simulink subsystem "Torque_Vectoring"  (R2023b)
settings: Solver=VariableStepAuto  StartTime=0.0  StopTime=10.0  RelTol=1e-3
undefined symbols (not defined in the file): chassis, powertrain, sim, suspension, tvs
libraries: simulink x1
settings Model: Creator=Inver  LastModifiedBy=Inver
settings SFSimCC: SimCustomHeaderCode="#include \"simplex.h\""  SimUserSources=Code_Generation_Project/simplex.c

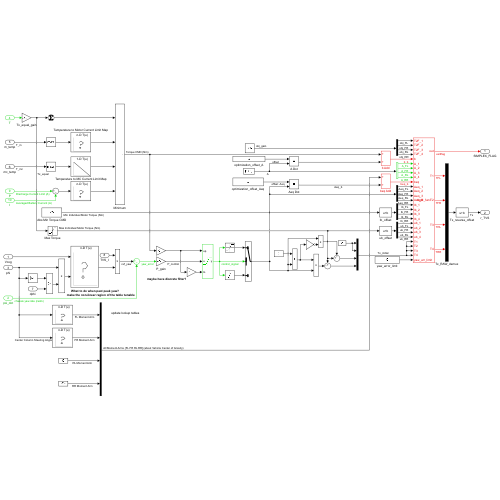
[thumbnail: Simulink's stored preview of the top-level diagram]
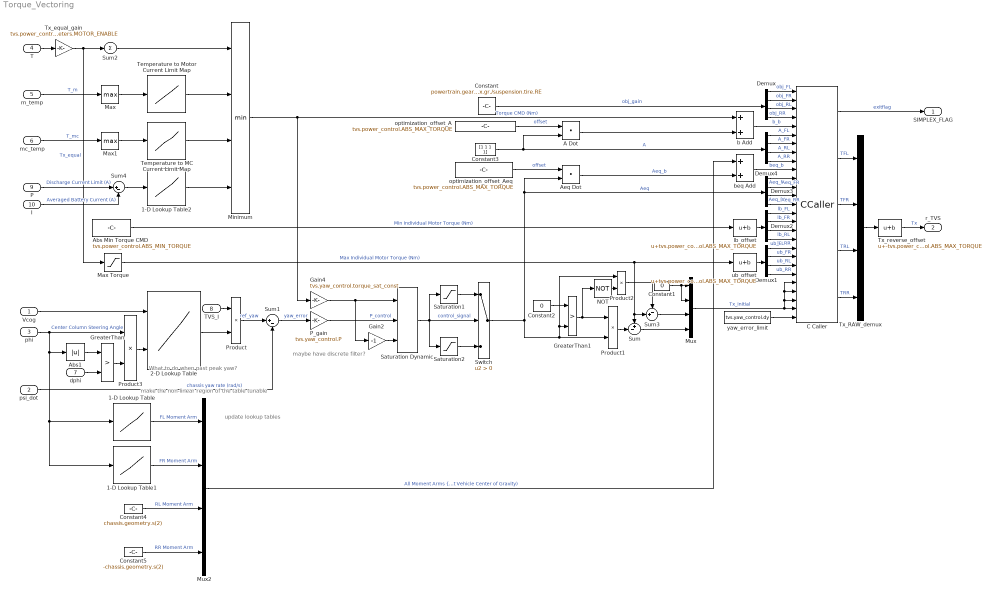
== system Torque_Vectoring ==
  note: make the non-linear region of the table tunable
  note: update lookup tables
  note: maybe have discrete filter?
  note: What to do when past peak yaw?
  Vcog : Inport
  psi_dot : Inport  Port=2  OutDataTypeStr=double  LockScale=on
  phi : Inport  Port=3
  T : Inport  Port=4  OutDataTypeStr=double  LockScale=on
  m_temp : Inport  Port=5
  mc_temp : Inport  Port=6
  dphi : Inport  Port=7
  TVS_I : Inport  Port=8
  P : Inport  Port=9  OutDataTypeStr=double  LockScale=on
  I : Inport  Port=10  OutDataTypeStr=double  LockScale=on
  1-D Lookup Table : Lookup_n-D  NumberOfTableDimensions=1  BreakpointsForDimension1=suspension.steering.theta_sweep  Table=suspension.steering.Aeq_left  ExtrapMethod=Clip  InternalRulePriority=Speed  RndMeth=Simplest
  1-D Lookup Table1 : Lookup_n-D  NumberOfTableDimensions=1  BreakpointsForDimension1=suspension.steering.theta_sweep  Table=suspension.steering.Aeq_right  ExtrapMethod=Clip  InternalRulePriority=Speed  RndMeth=Simplest
  1-D Lookup Table2 : Lookup_n-D  NumberOfTableDimensions=1  LookupTableObject=''  BreakpointsForDimension1=[5 0]  BreakpointsForDimension1FirstPoint=10  BreakpointsForDimension2FirstPoint=10  BreakpointsForDimension1Spacing=12  BreakpointsForDimension2Spacing=12  IndexSearchMethod=Evenly spaced points  Table=[tvs.power_control.ABS_MAX_TRQ_CMD 0]  InterpMethod=Flat  DiagnosticForOutOfRangeInput=Error  InternalRulePriority=Speed  RndMeth=Simplest
  2-D Lookup Table : Lookup_n-D  BreakpointsForDimension1=tvs.yaw_control.max_v_bp  BreakpointsForDimension2=[-fliplr(tvs.yaw_control.max_s_bp(2:end)) tvs.yaw_control.max_s_bp]  Table=[-flipud(tvs.yaw_control.max_yaw_table_ref(2:end,:)); tvs.yaw_control.max_yaw_table_ref]'  ExtrapMethod=Clip  InternalRulePriority=Speed  RndMeth=Simplest
      settings: InputPortMap=u0,u1
  A Dot : DotProduct  OutDataTypeStr=double
  Abs Min Torque CMD : Constant  Value=tvs.power_control.ABS_MIN_TORQUE  OutDataTypeStr=double
  Abs1 : Abs  SaturateOnIntegerOverflow=off
  Aeq Dot : DotProduct  OutDataTypeStr=double
  C Caller : CCaller  FunctionName=bigM_func  PortSpecificationStruct="%)30     .    N\"X   8    (     @         %    \"    !P    !     0         %  0 \"0    $    _    07)G3F%M90  4&]R=$YA;64 4V-O<&4     26YD97@     5'EP90      4VEZ90      27-';&]B86P   X    P    !@    @    $          4    (     0    ,    !         !   P!O=70 #@   #     &    \"     0         !0    @    !     P    $         $  # &]U=  .    .     8    (    !          %    \"     $    &     0         0  ...(+15750 chars)"
  Constant : Constant  Value=powertrain.gearbox.gr./suspension.tire.RE
  Constant1 : Constant  Value=0
  Constant2 : Constant  Value=0
  Constant3 : Constant  Value=[1 1 1 1]
  Constant4 : Constant  Value=chassis.geometry.s(2)  OutDataTypeStr=Inherit: Inherit via back propagation
  Constant5 : Constant  Value=-chassis.geometry.s(2)  OutDataTypeStr=Inherit: Inherit via back propagation
  Demux{,1..4} (5 alike) : Demux
  Gain2 : Gain  Gain=-1
  Gain4 : Gain  Gain=tvs.yaw_control.torque_sat_const
  GreaterThan : RelationalOperator  Operator=>  OutDataTypeStr=boolean  RndMeth=Simplest  InputSameDT=off
  GreaterThan1 : RelationalOperator  Operator=>  OutDataTypeStr=boolean  RndMeth=Simplest  InputSameDT=off
  Max : MinMax  Function=max
  Max Torque : Saturate  UpperLimit=tvs.power_control.ABS_MAX_TORQUE  LowerLimit=2.*tvs.power_control.dTx  OutDataTypeStr=Inherit: Inherit via back propagation
  Max1 : MinMax  Function=max
  Minimum : MinMax  Inputs=4
  Mux : Mux
  Mux2 : Mux
  NOT : Logic  Operator=NOT  IconShape=distinctive  AllPortsSameDT=off  OutDataTypeStr=boolean
  P_gain : Gain  Gain=tvs.yaw_control.P  ParamDataTypeStr=double  OutDataTypeStr=double
  Product : Product  OutDataTypeStr=Inherit: Inherit via back propagation
  Product1 : Product
  Product2 : Product
  Product3 : Product
  Saturation Dynamic : simulink/Discontinuities/Saturation Dynamic  OutMin=[]  OutMax=[]  OutDataTypeStr=Inherit: Same as second input  OutDataType=fixdt(1, 16)  OutScaling=2^-10  DoSatur=off
  Saturation1 : Saturate  UpperLimit=inf  LowerLimit=tvs.yaw_control.dB
  Saturation2 : Saturate  UpperLimit=-tvs.yaw_control.dB  LowerLimit=-inf
  Sum : Sum  Inputs=+-|
  Sum1 : Sum  Inputs=|+-  OutDataTypeStr=Inherit: Inherit via back propagation
  Sum2 : Sum  Inputs=+
  Sum3 : Sum  Inputs=-+|
  Sum4 : Sum  Inputs=|+-
  Switch : Switch  Criteria=u2 > Threshold  SaturateOnIntegerOverflow=off  InputSameDT=off
  Temperature to MC Current Limit Map : Lookup_n-D  NumberOfTableDimensions=1  BreakpointsForDimension1=[50 75]  IndexSearchMethod=Evenly spaced points  Table=[tvs.power_control.ABS_MAX_TRQ_CMD 0]  ExtrapMethod=Clip  UseLastTableValue=on  InternalRulePriority=Speed  RndMeth=Simplest
  Temperature to Motor Current Limit Map : Lookup_n-D  NumberOfTableDimensions=1  BreakpointsForDimension1=tvs.power_control.motor_t_bp  IndexSearchMethod=Evenly spaced points  Table=[tvs.power_control.ABS_MAX_TRQ_CMD 0]  ExtrapMethod=Clip  UseLastTableValue=on  InternalRulePriority=Speed  RndMeth=Simplest
  Tx_RAW_demux : Mux
  Tx_equal_gain : Gain  Gain=tvs.power_control.ABS_MAX_TORQUE.*sim.top_parameters.MOTOR_ENABLE  OutDataTypeStr=double
  Tx_reverse_offset : Bias  Bias=-tvs.power_control.ABS_MAX_TORQUE  SaturateOnIntegerOverflow=off
  b Add : Sum  OutDataTypeStr=double
  beq Add : Sum  OutDataTypeStr=double
  lb_offset : Bias  Bias=tvs.power_control.ABS_MAX_TORQUE  SaturateOnIntegerOverflow=off
  optimization_offset_A : Constant  Value=tvs.power_control.ABS_MAX_TORQUE  OutDataTypeStr=double
  optimization_offset_Aeq : Constant  Value=tvs.power_control.ABS_MAX_TORQUE  OutDataTypeStr=double
  ub_offset : Bias  Bias=tvs.power_control.ABS_MAX_TORQUE  SaturateOnIntegerOverflow=off
  yaw_error_limit : Constant  Value=tvs.yaw_control.dy  OutDataTypeStr=double
  SIMPLEX_FLAG : Outport
  r_TVS : Outport  Port=2
  wires:
  P_gain/1 -> Saturation Dynamic/2  "P_control"
  dphi/1 -> GreaterThan/2
  Gain4/1 -> Gain2/1, Saturation Dynamic/1
  Saturation2/1 -> Switch/3
  Gain2/1 -> Saturation Dynamic/3
  Sum1/1 -> P_gain/1  "yaw_error"
  Saturation1/1 -> Switch/1
  Abs1/1 -> GreaterThan/1
  GreaterThan/1 -> Product3/2
  2-D Lookup Table/1 -> Product/2
  Saturation Dynamic/1 -> Saturation1/1, Switch/2, Saturation2/1  "control_signal"
  psi_dot/1 -> Sum1/2  "chassis yaw rate (rad/s)"
  Product/1 -> Sum1/1  "ref_yaw"
  TVS_I/1 -> Product/1
  Max/1 -> Temperature to Motor Current Limit Map/1
  Temperature to MC Current Limit Map/1 -> Minimum/3
  Temperature to Motor Current Limit Map/1 -> Minimum/2
  Max1/1 -> Temperature to MC Current Limit Map/1
  mc_temp/1 -> Max1/1  "T_mc"
  Vcog/1 -> 2-D Lookup Table/1
  Minimum/1 -> Gain4/1, b Add/1  "Torque CMD (Nm)"
  Abs Min Torque CMD/1 -> lb_offset/1  "Min Individual Motor Torque (Nm)"
  Max Torque/1 -> ub_offset/1, Sum3/2, Sum/1  "Max Individual Motor Torque (Nm)"
  m_temp/1 -> Max/1  "T_m"
  beq Add/1 -> C Caller/10  "beq_b"
  Demux2/3 -> C Caller/17  "lb_RL"
  Demux3/1 -> C Caller/11  "Aeq_FL"
  Demux3/3 -> C Caller/13  "Aeq_RL"
  Demux2/4 -> C Caller/18  "lb_RR"
  Demux4/2 -> C Caller/7  "A_FR"
  A Dot/1 -> b Add/2
  Demux1/4 -> C Caller/22  "ub_RR"
  lb_offset/1 -> Demux2/1
  Constant/1 -> Demux/1  "obj_gain"
  yaw_error_limit/1 -> C Caller/27
  Demux2/1 -> C Caller/15  "lb_FL"
  Demux3/2 -> C Caller/12  "Aeq_FR"
  C Caller/5 -> Tx_RAW_demux/4  "TRR"
  Constant3/1 -> A Dot/2, Demux4/1  "A"
  Demux2/2 -> C Caller/16  "lb_FR"
  Demux/1 -> C Caller/1  "obj_FL"
  optimization_offset_Aeq/1 -> Aeq Dot/1  "offset"
  C Caller/4 -> Tx_RAW_demux/3  "TRL"
  C Caller/2 -> Tx_RAW_demux/1  "TFL"
  Demux3/4 -> C Caller/14  "Aeq_RR"
  Aeq Dot/1 -> beq Add/2  "Aeq_b"
  Demux4/4 -> C Caller/9  "A_RR"
  C Caller/3 -> Tx_RAW_demux/2  "TFR"
  Demux1/3 -> C Caller/21  "ub_RL"
  b Add/1 -> C Caller/5  "b_b"
  ub_offset/1 -> Demux1/1
  Demux1/2 -> C Caller/20  "ub_FR"
  Demux4/1 -> C Caller/6  "A_FL"
  Demux1/1 -> C Caller/19  "ub_FL"
  Demux/3 -> C Caller/3  "obj_RL"
  optimization_offset_A/1 -> A Dot/1  "offset"
  Demux4/3 -> C Caller/8  "A_RL"
  Demux/4 -> C Caller/4  "obj_RR"
  Switch/1 -> Product2/1, GreaterThan1/2, Product1/2, Aeq Dot/2, Demux3/1  "Aeq"
  Demux/2 -> C Caller/2  "obj_FR"
  Tx_equal_gain/1 -> Sum2/1, Max Torque/1  "Tx_equal"
  Tx_RAW_demux/1 -> Tx_reverse_offset/1
  Constant4/1 -> Mux2/3  "RL Moment Arm"
  Constant5/1 -> Mux2/4  "RR Moment Arm"
  phi/1 -> Product3/1, Abs1/1, 1-D Lookup Table1/1, 1-D Lookup Table/1  "Center Column Steering Angle"
  1-D Lookup Table/1 -> Mux2/1  "FL Moment Arm"
  1-D Lookup Table1/1 -> Mux2/2  "FR Moment Arm"
  Mux2/1 -> beq Add/1  "All Moment Arms {FL FR RL RR] (about Vehicle Center of Gravity)"
  T/1 -> Tx_equal_gain/1
  Sum2/1 -> Minimum/1
  Product3/1 -> 2-D Lookup Table/2
  P/1 -> Sum4/1  "Discharge Current Limit (A)"
  C Caller/1 -> SIMPLEX_FLAG/1  "exitflag"
  Tx_reverse_offset/1 -> r_TVS/1  "Tx"
  1-D Lookup Table2/1 -> Minimum/4
  NOT/1 -> Product2/2
  Product2/1 -> Sum3/1
  GreaterThan1/1 -> Product1/1, NOT/1
  Sum3/1 -> Mux/3
  Mux/1 -> C Caller/23, C Caller/24, C Caller/25, C Caller/26  "Tx_initial"
  Sum/1 -> Mux/4
  Product1/1 -> Sum/2
  Constant1/1 -> Mux/2, Mux/1
  Constant2/1 -> GreaterThan1/1
  I/1 -> Sum4/2  "Averaged Battery Current (A)"
  Sum4/1 -> 1-D Lookup Table2/1
